simulink model "Motor_ctrl_INST"  (R2025b)
settings: Solver=ode15s  StartTime=0.0  StopTime=1  FixedStep=Ts/10  MaxStep=Tstep  RelTol=1e-3  AbsTol=1e-3  EnableMultiTasking=on
InitFcn:
  | if ~exist('flagwp')
  |     tic
  |     init_sim
  | end
  | mex Motor_ctrl.c User_functions/Src/*.c
StopFcn:
  | if ~exist('flagwp')
  |   elapsed_time=toc
  | end
values from neighbouring files (symbols this model uses):
  accel = 5000    [init_sim.m]
  Bm = 0    [init_sim.m]
  Clarke_inv = [1 0;-0.5 sqrt(3)/2;-0.5 -sqrt(3)/2]    [init_sim.m]
  Ctrl_strategy = 1    [init_sim.m]
  Ctrl_type = 3    [init_sim.m]
  dem = 1    [init_sim.m]
  dT = motorModel.SyreDrive.Converter.dT * 1e-6    [init_sim.m]
  expC = motorModel.IronPMLossMap_dq.expC    [init_sim.m]
  expH = motorModel.IronPMLossMap_dq.expH    [init_sim.m]
  expPM = motorModel.IronPMLossMap_dq.expPM    [init_sim.m]
  Fd0 = interp2(motorModel.FluxMap_dq.Id,motorModel.FluxMap_dq.Iq,motorModel.FluxMap_dq.Fd,0,0)    [init_sim.m]
  Fm = interp2(Idd,Iqq,Fdd,0,0)    [init_sim.m]
  HS_ctrl = 1    [init_sim.m]
  Id_dqt = interpn(motorModel.FluxMapInv_dqt.dataF.Fd,motorModel.FluxMapInv_dqt.dataF.Fq,motorModel.FluxMapInv_dqt.dataF.th,motorModel.FluxMapInv_dqt.dataF.Id,Fd_dqt,Fq_dqt,th_dqt,'cubic')    [init_sim.m]
  Id_fe = motorModel.IronPMLossMap_dq.Id    [init_sim.m]
  InitIntg_d = Fm*cos(th0)    [init_sim.m]
  InitIntg_q = Fm*sin(th0)    [init_sim.m]
  inj_waveform = 1    [init_sim.m]
  Iq_dqt = interpn(motorModel.FluxMapInv_dqt.dataF.Fd,motorModel.FluxMapInv_dqt.dataF.Fq,motorModel.FluxMapInv_dqt.dataF.th,motorModel.FluxMapInv_dqt.dataF.Iq,Fd_dqt,Fq_dqt,th_dqt,'cubic')    [init_sim.m]
  Iq_fe = motorModel.IronPMLossMap_dq.Iq    [init_sim.m]
  IronLoss = 1    [init_sim.m]
  J = motorModel.data.J    [init_sim.m]
  n0 = motorModel.IronPMLossMap_dq.n0    [init_sim.m]
  p = motorModel.data.p    [init_sim.m]
  Pfe_c = motorModel.IronPMLossMap_dq.Pfes_c + motorModel.IronPMLossMap_dq.Pfer_c    [init_sim.m]
  Pfe_h = motorModel.IronPMLossMap_dq.Pfes_h + motorModel.IronPMLossMap_dq.Pfer_h    [init_sim.m]
  Ppm = motorModel.IronPMLossMap_dq.Ppm    [init_sim.m]
  Quad_Maps = 2    [init_sim.m]
  SS_on = 1    [init_sim.m]
  T_dqt = interpn(motorModel.FluxMapInv_dqt.dataF.Fd,motorModel.FluxMapInv_dqt.dataF.Fq,motorModel.FluxMapInv_dqt.dataF.th,motorModel.FluxMapInv_dqt.dataF.T,Fd_dqt,Fq_dqt,th_dqt,'cubic')    [init_sim.m]
  Tf = 0    [init_sim.m]
  th0 = 0    [init_sim.m]
  th_max = max(motorModel.FluxMapInv_dqt.dataF.th,[],'all')    [init_sim.m]
  th_min = min(motorModel.FluxMapInv_dqt.dataF.th,[],'all')    [init_sim.m]
  Ts = 1/motorModel.SyreDrive.Converter.fPWM    [init_sim.m]
  Tv = 0    [init_sim.m]
  VDC = motorModel.data.Vdc    [init_sim.m]
undefined symbols (not defined in the file or in its folder): ACloss, eMotor, fD_pu_norm, fD_vct_max, fD_vct_ref, fQ_pu_norm, fQ_vct_max, fQ_vct_ref, iD_pu_norm, idRef, interpn, iQ_pu_norm, iqRef, J_rot, magnitude, motorModelType, nRef, sigbuilder_block, T0
libraries: nesl_utility x43, fl_lib x41, ee_lib x8, simulink x8, eeTransforms x1
(part 2 of 4)

== system Motor_ctrl_INST/Power block - Inverter + Motor/Circuital/Inverter Model/Inverter Commands/Duty ==
  Dabc : Inport
  iABC : Inport  Port=2
  Demux : Demux  Outputs=3
  Gain : Gain  Gain=dT/Ts
  Mux14 : Mux  Inputs=6
  Sign : Signum
  Sum : Sum  Inputs=|+-
  X_d1 : Fcn  Expr=1-u(1)
  X_d12 : Fcn  Expr=1-u(1)
  X_d2 : Fcn  Expr=1-u(1)
  G : Outport  VectorParamsAs1DForOutWhenUnconnected=off
  wires:
  iABC/1 -> Sign/1
  Sign/1 -> Gain/1
  Demux/3 -> Mux14/5, X_d2/1
  X_d2/1 -> Mux14/6
  Demux/1 -> X_d12/1, Mux14/1
  Dabc/1 -> Sum/1
  Gain/1 -> Sum/2
  Sum/1 -> Demux/1
  Demux/2 -> Mux14/3, X_d1/1
  X_d1/1 -> Mux14/4
  X_d12/1 -> Mux14/2
  Mux14/1 -> G/1

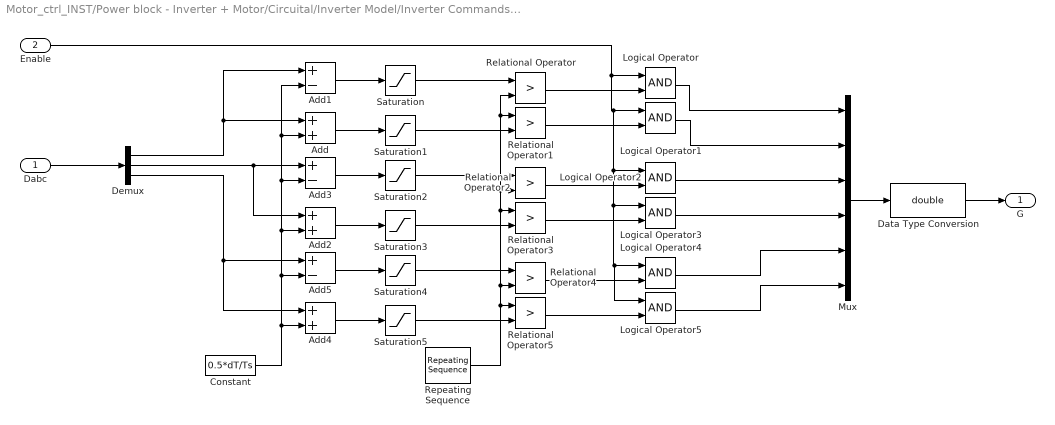
== system Motor_ctrl_INST/Power block - Inverter + Motor/Circuital/Inverter Model/Inverter Commands/PWM ==
  Dabc : Inport
  Enable : Inport  Port=2
  Add : Sum
  Add1 : Sum  Inputs=+-
  Add2 : Sum
  Add3 : Sum  Inputs=+-
  Add4 : Sum
  Add5 : Sum  Inputs=+-
  Constant : Constant  Value=0.5*dT/Ts
  Data Type Conversion : DataTypeConversion  OutDataTypeStr=double  SaturateOnIntegerOverflow=off  RndMeth=Floor
  Demux : Demux  Outputs=3
  Logical Operator{,1..5} (6 alike) : Logic  AllPortsSameDT=off  OutDataTypeStr=boolean
  Mux : Mux  Inputs=6
  Relational Operator{,1..5} (6 alike) : RelationalOperator  Operator=>  OutDataTypeStr=boolean  RndMeth=Simplest  InputSameDT=off
  Repeating Sequence : simulink/Sources/Repeating Sequence  rep_seq_t=[0 Ts/2 Ts]  rep_seq_y=[0 1 0]
  Saturation{,1..5} (6 alike) : Saturate  UpperLimit=1  LowerLimit=0
  G : Outport
  wires:
  Demux/3 -> Add4/1, Add5/1
  Add4/1 -> Saturation5/1
  Relational Operator4/1 -> Logical Operator4/2
  Add/1 -> Saturation1/1
  Relational Operator/1 -> Logical Operator/2
  Enable/1 -> Logical Operator5/1, Logical Operator4/1, Logical Operator3/1, Logical Operator2/1, Logical Operator1/1, Logical Operator/1
  Add5/1 -> Saturation4/1
  Relational Operator3/1 -> Logical Operator3/2
  Add1/1 -> Saturation/1
  Constant/1 -> Add1/2, Add/2, Add3/2, Add2/2, Add5/2, Add4/2
  Demux/1 -> Add1/1, Add/1
  Saturation2/1 -> Relational Operator2/1
  Demux/2 -> Add3/1, Add2/1
  Relational Operator2/1 -> Logical Operator2/2
  Saturation5/1 -> Relational Operator5/2
  Relational Operator1/1 -> Logical Operator1/2
  Add3/1 -> Saturation2/1
  Add2/1 -> Saturation3/1
  Saturation/1 -> Relational Operator/1
  Saturation4/1 -> Relational Operator4/1
  Saturation1/1 -> Relational Operator1/2
  Relational Operator5/1 -> Logical Operator5/2
  Logical Operator/1 -> Mux/1
  Saturation3/1 -> Relational Operator3/2
  Logical Operator1/1 -> Mux/2
  Dabc/1 -> Demux/1
  Mux/1 -> Data Type Conversion/1
  Logical Operator2/1 -> Mux/3
  Logical Operator3/1 -> Mux/4
  Logical Operator4/1 -> Mux/5
  Logical Operator5/1 -> Mux/6
  Repeating Sequence/1 -> Relational Operator/2, Relational Operator1/1, Relational Operator2/2, Relational Operator3/1, Relational Operator4/2, Relational Operator5/1
  Data Type Conversion/1 -> G/1

== system Motor_ctrl_INST/Power block - Inverter + Motor/Circuital/Motor model/CCG model/Mechanical equations ==
  Tload : Inport
  Tm : Inport  Port=2
  RPM : Inport  Port=3
  Constant : Constant  Value=Tf
  Constant1 : Constant  Value=Tv
  Delay One Step1 : Delay  DelayLength=1
  Delay One Step2 : Delay  DelayLength=1
  Gain1 : Gain  Gain=30/pi
  Gain2 : Gain  Gain=Bm  SaturateOnIntegerOverflow=on  OutDataTypeStr=Inherit: Same as input  ParamDataTypeStr=Inherit: Same as input
  Gain3 : Gain  Gain=1/J  SaturateOnIntegerOverflow=on  OutDataTypeStr=Inherit: Same as input  ParamDataTypeStr=Inherit: Same as input
  Gain4 : Gain  Gain=(2*pi)/60
  Integrator : Integrator  InitialCondition=th0  WrapState=on  WrappedStateUpperValue=2*pi  WrappedStateLowerValue=0
  Integrator1 : Integrator
  Integrator2 : Integrator  InitialCondition=th0  WrapState=on  WrappedStateUpperValue=2*pi  WrappedStateLowerValue=0
  Math Function1 : Math  Operator=magnitude^2  SignedPower=on
  Product : Product  SaturateOnIntegerOverflow=on  OutDataTypeStr=Inherit: Same as first input
  Product3 : Product  SaturateOnIntegerOverflow=on  OutDataTypeStr=Inherit: Same as first input
  Product6 : Product  SaturateOnIntegerOverflow=on  OutDataTypeStr=Inherit: Same as first input
  Sign : Signum  ZeroCross=off
  Sum1 : Sum  SaturateOnIntegerOverflow=on  OutDataTypeStr=Inherit: Same as first input
  Sum4 : Sum  SaturateOnIntegerOverflow=on  OutDataTypeStr=Inherit: Same as first input
  Sum5 : Sum  Inputs=--+  SaturateOnIntegerOverflow=on  OutDataTypeStr=Inherit: Same as first input
  Switch : Switch  Criteria=u2 > Threshold  Threshold=2.5  SaturateOnIntegerOverflow=off  InputSameDT=off
  Switch1 : Switch  Criteria=u2 > Threshold  Threshold=2.5  SaturateOnIntegerOverflow=off  InputSameDT=off
  n_m : Outport
  Pmec_out : Outport  Port=2  VectorParamsAs1DForOutWhenUnconnected=off
  thetar : Outport  Port=3
  wires:
  Gain3/1 -> Integrator1/1
  Gain2/1 -> Sum1/2
  Delay One Step2/1 -> Math Function1/1, Sign/1, Gain2/1
  Product6/1 -> Sum1/1
  Sum1/1 -> Sum5/2  "T mech loss"
  Tm/1 -> Delay One Step1/1
  Product/1 -> Pmec_out/1
  Tload/1 -> Sum5/1
  Math Function1/1 -> Product3/2
  Constant1/1 -> Product3/1
  Product3/1 -> Sum4/2
  Constant/1 -> Sum4/1
  Sum5/1 -> Gain3/1
  Sign/1 -> Product6/2
  Sum4/1 -> Product6/1
  Integrator2/1 -> Switch1/3
  Integrator/1 -> Switch1/1
  Switch1/1 -> thetar/1
  Switch/1 -> Gain1/1
  Integrator1/1 -> Integrator/1, Switch/1, Delay One Step2/1, Product/2
  Gain4/1 -> Switch/3, Integrator2/1
  [Ctrl_type] -> Switch/2, Switch1/2
  RPM/1 -> Gain4/1
  Delay One Step1/1 -> Sum5/3, Product/1
  Gain1/1 -> n_m/1

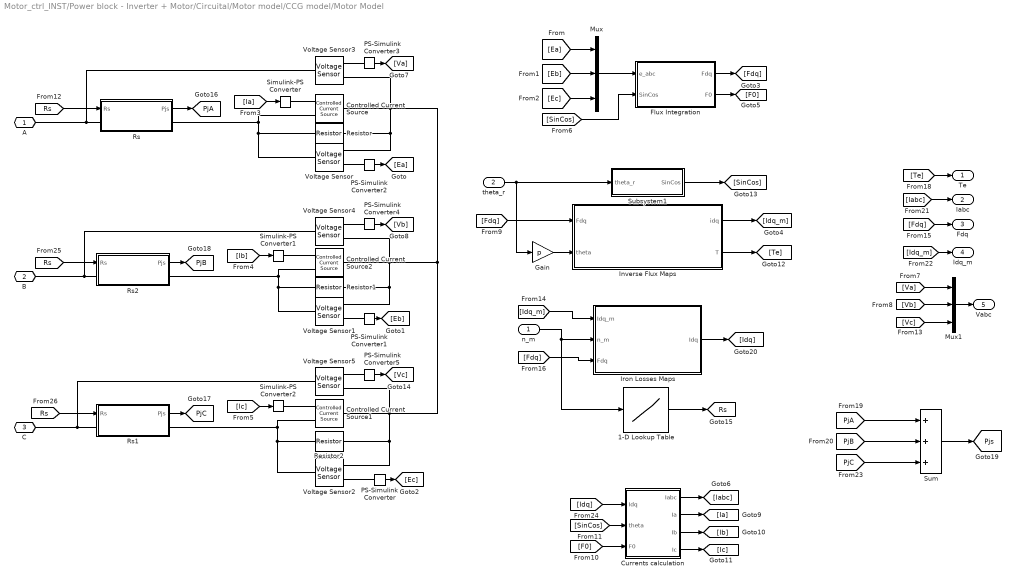
== system Motor_ctrl_INST/Power block - Inverter + Motor/Circuital/Motor model/CCG model/Motor Model ==
  n_m : Inport
  theta_r : Inport  Port=2
  1-D Lookup Table : Lookup_n-D  NumberOfTableDimensions=1  BreakpointsForDimension1=ACloss.n  Table=ACloss.Rac  InternalRulePriority=Speed  RndMeth=Simplest
  Controlled Current Source : fl_lib/Electrical/Electrical Sources/Controlled Current Source
  Controlled Current Source1 : fl_lib/Electrical/Electrical Sources/Controlled Current Source
  Controlled Current Source2 : fl_lib/Electrical/Electrical Sources/Controlled Current Source
  Currents calculation : Subsystem
  Flux Integration : Subsystem
  Gain : Gain  Gain=p
  Inverse Flux Maps : Subsystem  Variant=on
  Iron Losses Maps : Subsystem  Variant=on
  Mux : Mux  Inputs=3
  Mux1 : Mux  Inputs=3
  PS-Simulink Converter{,1..5} (6 alike) : nesl_utility/PS-Simulink Converter  PhysicalDomain=network_engine_domain  SubClassName=ps_output  LeftPortType=input  RightPortType=output  PseudoPeriodic=off  Frequencies=[]  VectorFormat=1-D array  Unit=inherit  AffineConversion=off
  Resistor : ee_lib/Passive/Resistor  R=1e9 Ohm  enable_R_tol=0  R_tol=5  tol_distribution=1  nSigma=4  enable_operating_limits=0  operating_limit_action=2  power_rating=1 W  max_working_voltage=100 V  noise_mode=0  Tdevice=25 degC  sample_time=1e-3 s  repeatability=1  user_seed=0  auto_seed=4111000739  power_derating_T1=70 degC  power_derating_T2=155 degC  operating_temperature_range_vec=[-50, 150] degC  alpha=3.93e-3 1/K  Tmeas=25 degC  thermal_mass=100 J/K  temperature_specify=off  temperature_priority=High  temperature=298.15 K  temperature_nominal_specify=off  temperature_nominal_value=1  temperature_nominal_unit=K
  Resistor1 : ee_lib/Passive/Resistor  R=1e9 Ohm  enable_R_tol=0  R_tol=5  tol_distribution=1  nSigma=4  enable_operating_limits=0  operating_limit_action=2  power_rating=1 W  max_working_voltage=100 V  noise_mode=0  Tdevice=25 degC  sample_time=1e-3 s  repeatability=1  user_seed=0  auto_seed=2084672538  power_derating_T1=70 degC  power_derating_T2=155 degC  operating_temperature_range_vec=[-50, 150] degC  alpha=3.93e-3 1/K  Tmeas=25 degC  thermal_mass=100 J/K  temperature_specify=off  temperature_priority=High  temperature=298.15 K  temperature_nominal_specify=off  temperature_nominal_value=1  temperature_nominal_unit=K
  Resistor2 : ee_lib/Passive/Resistor  R=1e9 Ohm  enable_R_tol=0  R_tol=5  tol_distribution=1  nSigma=4  enable_operating_limits=0  operating_limit_action=2  power_rating=1 W  max_working_voltage=100 V  noise_mode=0  Tdevice=25 degC  sample_time=1e-3 s  repeatability=1  user_seed=0  auto_seed=3437178441  power_derating_T1=70 degC  power_derating_T2=155 degC  operating_temperature_range_vec=[-50, 150] degC  alpha=3.93e-3 1/K  Tmeas=25 degC  thermal_mass=100 J/K  temperature_specify=off  temperature_priority=High  temperature=298.15 K  temperature_nominal_specify=off  temperature_nominal_value=1  temperature_nominal_unit=K
  Rs : Subsystem  Variant=on
  Rs1 : Subsystem  Variant=on
  Rs2 : Subsystem  Variant=on
  Simulink-PS Converter : nesl_utility/Simulink-PS Converter  PhysicalDomain=network_engine_domain  SubClassName=ps_input  LeftPortType=input  RightPortType=output  PseudoPeriodic=off  Frequencies=[]  NoiseDistribution=none  NoiseParameters=[]  Unit=1  AffineConversion=off  FilteringAndDerivatives=provide  SimscapeFilterOrder=1  InputFilterTimeConstant=0.001  UdotUserProvided=0
  Simulink-PS Converter1 : nesl_utility/Simulink-PS Converter  PhysicalDomain=network_engine_domain  SubClassName=ps_input  LeftPortType=input  RightPortType=output  PseudoPeriodic=off  Frequencies=[]  NoiseDistribution=none  NoiseParameters=[]  Unit=1  AffineConversion=off  FilteringAndDerivatives=provide  SimscapeFilterOrder=1  InputFilterTimeConstant=0.001  UdotUserProvided=0
  Simulink-PS Converter2 : nesl_utility/Simulink-PS Converter  PhysicalDomain=network_engine_domain  SubClassName=ps_input  LeftPortType=input  RightPortType=output  PseudoPeriodic=off  Frequencies=[]  NoiseDistribution=none  NoiseParameters=[]  Unit=1  AffineConversion=off  FilteringAndDerivatives=provide  SimscapeFilterOrder=1  InputFilterTimeConstant=0.001  UdotUserProvided=0
  Subsystem1 : Subsystem
  Sum : Sum  Inputs=+++
  Voltage Sensor{,1..5} (6 alike) : fl_lib/Electrical/Electrical Sensors/Voltage Sensor
  A : PMIOPort  Side=Left
  B : PMIOPort  Port=2  Side=Left
  C : PMIOPort  Port=3  Side=Left
  Te : Outport
  Iabc : Outport  Port=2
  Fdq : Outport  Port=3
  Idq_m : Outport  Port=4
  Vabc : Outport  Port=5
  tag scope: PjA=global, PjB=global, PjC=global, Pjs=global, Rs=global
  wires:
  PS-Simulink Converter2/1 -> [Ea]
  PS-Simulink Converter1/1 -> [Eb]
  PS-Simulink Converter/1 -> [Ec]
  [Ea] -> Mux/1
  [Eb] -> Mux/2
  [Ec] -> Mux/3
  [Ia] -> Simulink-PS Converter/1
  [Ib] -> Simulink-PS Converter1/1
  [Ic] -> Simulink-PS Converter2/1
  Inverse Flux Maps/1(idq) -> [Idq_m]
  [Iabc] -> Iabc/1
  [Idq_m] -> Idq_m/1
  [F0] -> Currents calculation/3(F0)
  [SinCos] -> Currents calculation/2(theta)
  [Idq] -> Currents calculation/1(Idq)
  [Fdq] -> Inverse Flux Maps/1(Fdq)
  [Te] -> Te/1
  theta_r/1 -> Gain/1, Subsystem1/1(theta_r)
  Currents calculation/1(Iabc) -> [Iabc]
  [Fdq] -> Fdq/1
  Subsystem1/1(SinCos) -> [SinCos]
  Mux/1 -> Flux Integration/1(e_abc)
  Flux Integration/1(Fdq) -> [Fdq]
  [SinCos] -> Flux Integration/2(SinCos)
  Flux Integration/2(F0) -> [F0]
  PS-Simulink Converter3/1 -> [Va]
  PS-Simulink Converter4/1 -> [Vb]
  PS-Simulink Converter5/1 -> [Vc]
  [Va] -> Mux1/1
  [Vb] -> Mux1/2
  [Vc] -> Mux1/3
  Mux1/1 -> Vabc/1
  Inverse Flux Maps/2(T) -> [Te]
  n_m/1 -> 1-D Lookup Table/1, Iron Losses Maps/2(n_m)
  [Fdq] -> Iron Losses Maps/3(Fdq)
  [Idq_m] -> Iron Losses Maps/1(Idq_m)
  Iron Losses Maps/1(Idq) -> [Idq]
  Currents calculation/2(Ia) -> [Ia]
  Currents calculation/3(Ib) -> [Ib]
  Currents calculation/4(Ic) -> [Ic]
  Gain/1 -> Inverse Flux Maps/2(theta)
  1-D Lookup Table/1 -> [Rs]
  [Rs] -> Rs/1(Rs)
  Rs/1(Pjs) -> [PjA]
  Rs2/1(Pjs) -> [PjB]
  Rs1/1(Pjs) -> [PjC]
  Sum/1 -> [Pjs]
  [PjC] -> Sum/3
  [PjB] -> Sum/2
  [PjA] -> Sum/1
  [Rs] -> Rs2/1(Rs)
  [Rs] -> Rs1/1(Rs)
  connections:
  Controlled Current Source/LConn1 -- Voltage Sensor3/RConn2 -- Voltage Sensor5/RConn2 -- Voltage Sensor2/RConn2 -- Resistor2/RConn1 -- Controlled Current Source1/LConn1 -- Voltage Sensor4/RConn2 -- Voltage Sensor1/RConn2 -- Resistor1/RConn1 -- Controlled Current Source2/LConn1 -- Voltage Sensor/RConn2 -- Resistor/RConn1
  Simulink-PS Converter/RConn1 -- Controlled Current Source/RConn1
  Simulink-PS Converter1/RConn1 -- Controlled Current Source2/RConn1
  Simulink-PS Converter2/RConn1 -- Controlled Current Source1/RConn1
  PS-Simulink Converter/LConn1 -- Voltage Sensor2/RConn1
  PS-Simulink Converter1/LConn1 -- Voltage Sensor1/RConn1
  PS-Simulink Converter2/LConn1 -- Voltage Sensor/RConn1
  Voltage Sensor2/LConn1 -- Resistor2/LConn1 -- Rs1/RConn1 -- Controlled Current Source1/RConn2
  Resistor1/LConn1 -- Rs2/RConn1 -- Controlled Current Source2/RConn2 -- Voltage Sensor1/LConn1
  Resistor/LConn1 -- Voltage Sensor/LConn1 -- Controlled Current Source/RConn2 -- Rs/RConn1
  Voltage Sensor3/LConn1 -- Rs/LConn1 -- A/RConn1
  Voltage Sensor4/LConn1 -- B/RConn1 -- Rs2/LConn1
  Voltage Sensor5/LConn1 -- Rs1/LConn1 -- C/RConn1
  Voltage Sensor3/RConn1 -- PS-Simulink Converter3/LConn1
  Voltage Sensor4/RConn1 -- PS-Simulink Converter4/LConn1
  Voltage Sensor5/RConn1 -- PS-Simulink Converter5/LConn1

== system Motor_ctrl_INST/Power block - Inverter + Motor/Circuital/Motor model/SimScape FEM-based PMSM/Load model ==
  note: 1) Add Subsystem or Model blocks as valid variant choices.
      | 2) You cannot connect blocks at this level. At simulation, connectivity is automatically
      | determined, based on the active variant and port name matching.
  T_ref : Inport
  n_ref : Inport  Port=2
  Ideal speed load : Subsystem  VariantControl=Ctrl_type<2.5
  Ideal torque load : Subsystem  VariantControl=Ctrl_type>2.5
  R : PMIOPort  Side=Left
  C : PMIOPort  Port=2  Side=Left

== system Motor_ctrl_INST/Power block - Inverter + Motor/Circuital/Motor model/SimScape FEM-based PMSM/abc2dq ==
  Xabc : Inport
  theta_r : Inport  Port=2
  Bus Creator : BusCreator  Inputs=2
  Demux : Demux  Outputs=3
  Subsystem1 : Subsystem
  Terminator : Terminator
  ab->dq : Subsystem
      mask Display: disp('A(-theta)')
  abc->ab0 : Subsystem
  X_dq : Outport
  wires:
  ab->dq/1(X_dq) -> X_dq/1
  Xabc/1 -> abc->ab0/1(eabc)
  Demux/1 -> Bus Creator/1
  Demux/2 -> Bus Creator/2
  abc->ab0/1(eab0) -> Demux/1
  Bus Creator/1 -> ab->dq/1(X_ab)
  Subsystem1/1(SinCos) -> ab->dq/2(sin,cos)
  theta_r/1 -> Subsystem1/1(theta_r)
  Demux/3 -> Terminator/1

== system Motor_ctrl_INST/Power block - Inverter + Motor/Circuital/Motor model/SimScape FEM-based PMSM/abc2dq1 ==
  Xabc : Inport
  theta_r : Inport  Port=2
  Bus Creator : BusCreator  Inputs=2
  Demux : Demux  Outputs=3
  Subsystem1 : Subsystem
  Terminator : Terminator
  ab->dq : Subsystem
      mask Display: disp('A(-theta)')
  abc->ab0 : Subsystem
  X_dq : Outport
  wires:
  ab->dq/1(X_dq) -> X_dq/1
  Xabc/1 -> abc->ab0/1(eabc)
  Demux/1 -> Bus Creator/1
  Demux/2 -> Bus Creator/2
  abc->ab0/1(eab0) -> Demux/1
  Bus Creator/1 -> ab->dq/1(X_ab)
  Subsystem1/1(SinCos) -> ab->dq/2(sin,cos)
  theta_r/1 -> Subsystem1/1(theta_r)
  Demux/3 -> Terminator/1

== system Motor_ctrl_INST/Power block - Inverter + Motor/Noncircuital/FM/Motor Model/Inverse Flux Maps ==
  note: 1) Add Subsystem or Model blocks as valid variant choices.
      | 2) You cannot connect blocks at this level. At simulation, connectivity is automatically
      | determined, based on the active variant and port name matching.
  Vabc : Inport
  theta_elt : Inport  Port=2
  n : Inport  Port=3
  2D LUT : Subsystem  VariantControl=FMapsModel==1
  3D LUTs : Subsystem  VariantControl=FMapsModel==-1
  idq : Outport
  T : Outport  Port=2
  i0 : Outport  Port=3
  Fdq : Outport  Port=4

== system Motor_ctrl_INST/Power block - Inverter + Motor/Noncircuital/FM/Motor Model/Iron Losses Maps ==
  note: 1) Add Subsystem or Model blocks as valid variant choices.
      | 2) You cannot connect blocks at this level. At simulation, connectivity is automatically
      | determined, based on the active variant and port name matching.
  Idq_m : Inport
  n_m : Inport  Port=2
  Fdq : Inport  Port=3
  T_m : Inport  Port=4
  Iron Losses : Subsystem  VariantControl=IronLoss==1
  No Iron Losses : Subsystem  VariantControl=IronLoss==0
  Idq : Outport

== system Motor_ctrl_INST/Power block - Inverter + Motor/Noncircuital/Inverter Model/Inverter Commands/Duty ==
  Dabc : Inport
  iABC : Inport  Port=2
  Gain : Gain  Gain=dT/Ts
  Gain1 : Gain  Gain=2*VDC/3
  Mux2 : Mux  Inputs=3
  Sign : Signum
  Sum : Sum  Inputs=|+-
  Unit Delay : UnitDelay  SampleTime=-1  HasFrameUpgradeWarning=on
  X_d6 : Fcn  Expr=-0.5*u(1) + u(2) - 0.5*u(3)
  X_d7 : Fcn  Expr=u(1) - 0.5*u(2) - 0.5*u(3)
  X_d8 : Fcn  Expr=-0.5*u(1) - 0.5*u(2) + u(3)
  Vabc : Outport  VectorParamsAs1DForOutWhenUnconnected=off
  wires:
  iABC/1 -> Sign/1
  Sign/1 -> Gain/1
  Dabc/1 -> Sum/1
  Gain/1 -> Sum/2
  Sum/1 -> Gain1/1
  X_d7/1 -> Mux2/1
  X_d6/1 -> Mux2/2
  X_d8/1 -> Mux2/3
  Unit Delay/1 -> Vabc/1
  Mux2/1 -> Unit Delay/1
  Gain1/1 -> X_d6/1, X_d8/1, X_d7/1

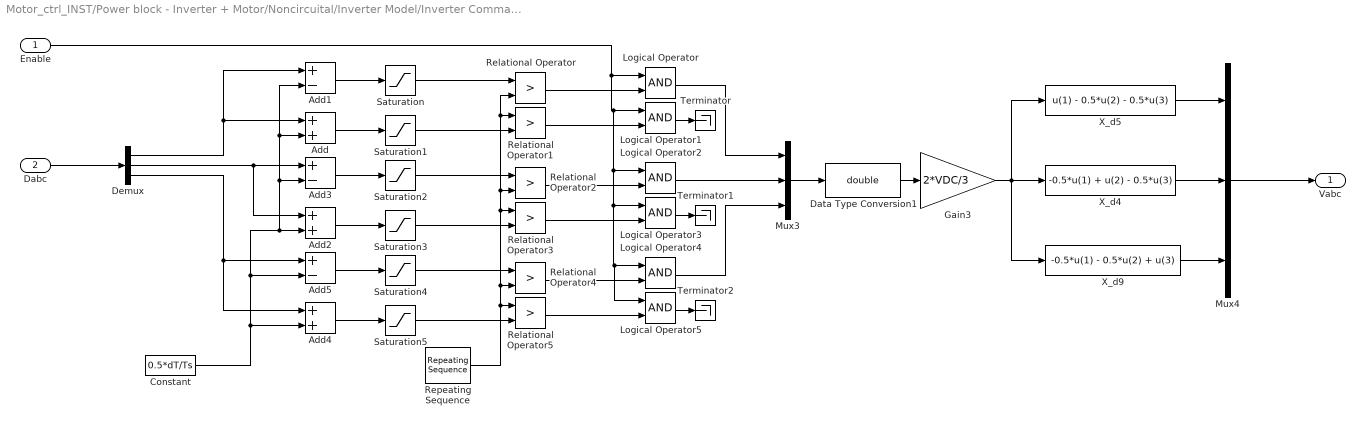
== system Motor_ctrl_INST/Power block - Inverter + Motor/Noncircuital/Inverter Model/Inverter Commands/PWM ==
  Enable : Inport
  Dabc : Inport  Port=2
  Add : Sum
  Add1 : Sum  Inputs=+-
  Add2 : Sum
  Add3 : Sum  Inputs=+-
  Add4 : Sum
  Add5 : Sum  Inputs=+-
  Constant : Constant  Value=0.5*dT/Ts
  Data Type Conversion1 : DataTypeConversion  OutDataTypeStr=double  SaturateOnIntegerOverflow=off  RndMeth=Floor
  Demux : Demux  Outputs=3
  Gain3 : Gain  Gain=2*VDC/3
  Logical Operator{,1..5} (6 alike) : Logic  AllPortsSameDT=off  OutDataTypeStr=boolean
  Mux3 : Mux  Inputs=3
  Mux4 : Mux  Inputs=3
  Relational Operator{,1..5} (6 alike) : RelationalOperator  Operator=>  OutDataTypeStr=boolean  RndMeth=Simplest  InputSameDT=off
  Repeating Sequence : simulink/Sources/Repeating Sequence  rep_seq_t=[0 Ts/2 Ts]  rep_seq_y=[0 1 0]
  Saturation{,1..5} (6 alike) : Saturate  UpperLimit=1  LowerLimit=0
  Terminator : Terminator
  Terminator1 : Terminator
  Terminator2 : Terminator
  X_d4 : Fcn  Expr=-0.5*u(1) + u(2) - 0.5*u(3)
  X_d5 : Fcn  Expr=u(1) - 0.5*u(2) - 0.5*u(3)
  X_d9 : Fcn  Expr=-0.5*u(1) - 0.5*u(2) + u(3)
  Vabc : Outport
  wires:
  Demux/3 -> Add4/1, Add5/1
  Add4/1 -> Saturation5/1
  Relational Operator4/1 -> Logical Operator4/2
  Add/1 -> Saturation1/1
  Relational Operator/1 -> Logical Operator/2
  Enable/1 -> Logical Operator5/1, Logical Operator4/1, Logical Operator3/1, Logical Operator2/1, Logical Operator1/1, Logical Operator/1
  Add5/1 -> Saturation4/1
  Relational Operator3/1 -> Logical Operator3/2
  Add1/1 -> Saturation/1
  Demux/1 -> Add1/1, Add/1
  Saturation2/1 -> Relational Operator2/1
  Demux/2 -> Add3/1, Add2/1
  Relational Operator2/1 -> Logical Operator2/2
  Saturation5/1 -> Relational Operator5/2
  Relational Operator1/1 -> Logical Operator1/2
  Add3/1 -> Saturation2/1
  Add2/1 -> Saturation3/1
  Saturation/1 -> Relational Operator/1
  Saturation4/1 -> Relational Operator4/1
  Saturation1/1 -> Relational Operator1/2
  Relational Operator5/1 -> Logical Operator5/2
  Logical Operator/1 -> Mux3/1
  Saturation3/1 -> Relational Operator3/2
  Logical Operator2/1 -> Mux3/2
  Logical Operator4/1 -> Mux3/3
  Repeating Sequence/1 -> Relational Operator/2, Relational Operator1/1, Relational Operator2/2, Relational Operator3/1, Relational Operator4/2, Relational Operator5/1
  X_d4/1 -> Mux4/2
  X_d5/1 -> Mux4/1
  X_d9/1 -> Mux4/3
  Gain3/1 -> X_d9/1, X_d5/1, X_d4/1
  Mux3/1 -> Data Type Conversion1/1
  Data Type Conversion1/1 -> Gain3/1
  Constant/1 -> Add1/2, Add/2, Add3/2, Add2/2, Add5/2, Add4/2
  Dabc/1 -> Demux/1
  Mux4/1 -> Vabc/1
  Logical Operator1/1 -> Terminator/1
  Logical Operator3/1 -> Terminator1/1
  Logical Operator5/1 -> Terminator2/1

== system Motor_ctrl_INST/Power block - Inverter + Motor/Circuital/Motor model/CCG model/Motor Model/Currents calculation ==
  Idq : Inport
  theta : Inport  Port=2
  F0 : Inport  Port=3
  2-->3 : Gain  Gain=Clarke_inv  Multiplication=Matrix(K*u)  SaturateOnIntegerOverflow=on  OutDataTypeStr=Inherit: Same as input  ParamDataTypeStr=Inherit: Same as input
  Demux : Demux  Outputs=3
  Demux1 : Demux  Outputs=3
  Gain1 : Gain  Gain=0
  Gain2 : Gain  Gain=1/3
  Mux3 : Mux  Inputs=3
  Sum1 : Sum  Inputs=|++
  Sum2 : Sum  Inputs=|++
  Sum3 : Sum  Inputs=|++
  dq->ab1 : Subsystem
      mask Display: disp('A(theta)')
  Iabc : Outport
  Ia : Outport  Port=2
  Ib : Outport  Port=3
  Ic : Outport  Port=4
  wires:
  Sum2/1 -> Mux3/2
  Demux1/3 -> Sum3/1
  2-->3/1 -> Demux1/1
  Demux1/1 -> Sum1/1
  Demux1/2 -> Sum2/1
  F0/1 -> Gain1/1
  Sum1/1 -> Mux3/1
  Sum3/1 -> Mux3/3
  Mux3/1 -> Demux/1, Iabc/1
  Gain1/1 -> Gain2/1
  Gain2/1 -> Sum1/2, Sum2/2, Sum3/2
  Idq/1 -> dq->ab1/1(X_ab)
  theta/1 -> dq->ab1/2(sin,cos)
  dq->ab1/1(X_dq) -> 2-->3/1
  Demux/1 -> Ia/1
  Demux/2 -> Ib/1
  Demux/3 -> Ic/1

== system Motor_ctrl_INST/Power block - Inverter + Motor/Circuital/Motor model/CCG model/Motor Model/Flux Integration ==
  e_abc : Inport
  SinCos : Inport  Port=2
  Demux : Demux  Outputs=3
  Demux1 : Demux  Outputs=3
  Integrator1 : Integrator  InitialCondition=InitIntg_d
  Integrator4 : Integrator  InitialCondition=InitIntg_q
  Integrator5 : Integrator
  Mux : Mux  Inputs=3
  Mux1 : Mux  Inputs=2
  ab->dq : Subsystem
      mask Display: disp('A(-theta)')
  abc->ab0 : Subsystem
  Fdq : Outport
  F0 : Outport  Port=2
  wires:
  Demux/3 -> Integrator5/1
  Demux/2 -> Integrator4/1
  Demux/1 -> Integrator1/1
  Integrator4/1 -> Mux/2
  Integrator1/1 -> Mux/1
  Integrator5/1 -> Mux/3
  e_abc/1 -> abc->ab0/1(eabc)
  abc->ab0/1(eab0) -> Demux/1
  Demux1/2 -> Mux1/2
  Mux1/1 -> ab->dq/1(X_ab)
  Demux1/1 -> Mux1/1
  ab->dq/1(X_dq) -> Fdq/1
  Demux1/3 -> F0/1
  SinCos/1 -> ab->dq/2(sin,cos)
  Mux/1 -> Demux1/1

== system Motor_ctrl_INST/Power block - Inverter + Motor/Circuital/Motor model/CCG model/Motor Model/Inverse Flux Maps ==
  note: 1) Add Subsystem or Model blocks as valid variant choices.
      | 2) You cannot connect blocks at this level. At simulation, connectivity is automatically
      | determined, based on the active variant and port name matching.
  Fdq : Inport
  theta : Inport  Port=2
  2D LUT : Subsystem  VariantControl=FMapsModel==1
  3D LUTs : Subsystem  VariantControl=FMapsModel==-1
  idq : Outport
  T : Outport  Port=2

== system Motor_ctrl_INST/Power block - Inverter + Motor/Circuital/Motor model/CCG model/Motor Model/Iron Losses Maps ==
  note: 1) Add Subsystem or Model blocks as valid variant choices.
      | 2) You cannot connect blocks at this level. At simulation, connectivity is automatically
      | determined, based on the active variant and port name matching.
  Idq_m : Inport
  n_m : Inport  Port=2
  Fdq : Inport  Port=3
  Iron Losses : Subsystem  VariantControl=IronLoss==1
  No Iron Losses : Subsystem  VariantControl=IronLoss==0
  Idq : Outport

== system Motor_ctrl_INST/Power block - Inverter + Motor/Circuital/Motor model/CCG model/Motor Model/Rs ==
  note: 1) Add Subsystem or Model blocks as valid variant choices.
      | 2) You cannot connect blocks at this level. At simulation, connectivity is automatically
      | determined, based on the active variant and port name matching.
  Rs : Inport
  no AC loss : Subsystem  VariantControl=ACloss.enable==0
  yes AC loss : Subsystem  VariantControl=ACloss.enable==1
  In : PMIOPort  Side=Left
  Out : PMIOPort  Port=2  Side=Right
  Pjs : Outport

== system Motor_ctrl_INST/Power block - Inverter + Motor/Circuital/Motor model/CCG model/Motor Model/Rs1 ==
  note: 1) Add Subsystem or Model blocks as valid variant choices.
      | 2) You cannot connect blocks at this level. At simulation, connectivity is automatically
      | determined, based on the active variant and port name matching.
  Rs : Inport
  no AC loss : Subsystem  VariantControl=ACloss.enable==0
  yes AC loss : Subsystem  VariantControl=ACloss.enable==1
  In : PMIOPort  Side=Left
  Out : PMIOPort  Port=2  Side=Right
  Pjs : Outport

== system Motor_ctrl_INST/Power block - Inverter + Motor/Circuital/Motor model/CCG model/Motor Model/Rs2 ==
  note: 1) Add Subsystem or Model blocks as valid variant choices.
      | 2) You cannot connect blocks at this level. At simulation, connectivity is automatically
      | determined, based on the active variant and port name matching.
  Rs : Inport
  no AC loss : Subsystem  VariantControl=ACloss.enable==0
  yes AC loss : Subsystem  VariantControl=ACloss.enable==1
  In : PMIOPort  Side=Left
  Out : PMIOPort  Port=2  Side=Right
  Pjs : Outport

== system Motor_ctrl_INST/Power block - Inverter + Motor/Circuital/Motor model/CCG model/Motor Model/Subsystem1 ==
  theta_r : Inport
  Gain1 : Gain  Gain=p
  Mux3 : Mux  Inputs=2
  Scope : Scope
  Scope1 : Scope
  Sin : Trigonometry
  Sin1 : Trigonometry  Operator=cos
  SinCos : Outport
  wires:
  Sin1/1 -> Mux3/2
  Sin/1 -> Mux3/1
  Mux3/1 -> Scope/1, SinCos/1
  Gain1/1 -> Scope1/1, Sin/1, Sin1/1
  theta_r/1 -> Gain1/1

== system Motor_ctrl_INST/Power block - Inverter + Motor/Circuital/Motor model/SimScape FEM-based PMSM/Load model/Ideal speed load ==
  T_ref : Inport
  n_ref : Inport  Port=2
  Gain : Gain  Gain=pi/30
  Ideal Angular Velocity Source : fl_lib/Mechanical/Mechanical Sources/Ideal Angular Velocity Source
  Simulink-PS Converter : nesl_utility/Simulink-PS Converter  PhysicalDomain=network_engine_domain  SubClassName=ps_input  LeftPortType=input  RightPortType=output  PseudoPeriodic=off  Frequencies=[]  NoiseDistribution=none  NoiseParameters=[]  Unit=1  AffineConversion=off  FilteringAndDerivatives=filter  SimscapeFilterOrder=1  InputFilterTimeConstant=0.001  UdotUserProvided=0
  Terminator : Terminator
  R : PMIOPort  Side=Left
  C : PMIOPort  Port=2  Side=Left
  wires:
  Gain/1 -> Simulink-PS Converter/1
  n_ref/1 -> Gain/1
  T_ref/1 -> Terminator/1
  connections:
  Ideal Angular Velocity Source/LConn1 -- R/RConn1
  Ideal Angular Velocity Source/RConn2 -- C/RConn1
  Simulink-PS Converter/RConn1 -- Ideal Angular Velocity Source/RConn1

== system Motor_ctrl_INST/Power block - Inverter + Motor/Circuital/Motor model/SimScape FEM-based PMSM/Load model/Ideal torque load ==
  T_ref : Inport
  n_ref : Inport  Port=2
  Ideal Torque Source : fl_lib/Mechanical/Mechanical Sources/Ideal Torque Source
  Simulink-PS Converter : nesl_utility/Simulink-PS Converter  PhysicalDomain=network_engine_domain  SubClassName=ps_input  LeftPortType=input  RightPortType=output  PseudoPeriodic=off  Frequencies=[]  NoiseDistribution=none  NoiseParameters=[]  Unit=1  AffineConversion=off  FilteringAndDerivatives=provide  SimscapeFilterOrder=1  InputFilterTimeConstant=0.001  UdotUserProvided=0
  Terminator : Terminator
  R : PMIOPort  Side=Left
  C : PMIOPort  Port=2  Side=Left
  wires:
  n_ref/1 -> Terminator/1
  T_ref/1 -> Simulink-PS Converter/1
  connections:
  Ideal Torque Source/LConn1 -- R/RConn1
  Ideal Torque Source/RConn2 -- C/RConn1
  Simulink-PS Converter/RConn1 -- Ideal Torque Source/RConn1

== system Motor_ctrl_INST/Power block - Inverter + Motor/Circuital/Motor model/SimScape FEM-based PMSM/abc2dq/Subsystem1 ==
  theta_r : Inport
  Gain1 : Gain  Gain=p
  Mux3 : Mux  Inputs=2
  Scope : Scope
  Scope1 : Scope
  Sin : Trigonometry
  Sin1 : Trigonometry  Operator=cos
  SinCos : Outport
  wires:
  Sin1/1 -> Mux3/2
  Sin/1 -> Mux3/1
  Mux3/1 -> Scope/1, SinCos/1
  Gain1/1 -> Scope1/1, Sin/1, Sin1/1
  theta_r/1 -> Gain1/1

== system Motor_ctrl_INST/Power block - Inverter + Motor/Circuital/Motor model/SimScape FEM-based PMSM/abc2dq/ab->dq ==
  X_ab : Inport
  sin,cos : Inport  Port=2
  Demux : Demux  Outputs=2
  Demux1 : Demux  Outputs=2
  Mux : Mux  Commented=on  Inputs=2
  Mux1 : Mux  Commented=on  Inputs=2
  Mux2 : Mux  Inputs=2
  Product{,1..3} (4 alike) : Product
  Subtract : Sum
  Subtract1 : Sum  Inputs=-+
  X_d : Fcn  Commented=on  Expr=u(1)*u(4) + u(2)*u(3)
  X_q : Fcn  Commented=on  Expr=- u(1)*u(3) + u(2)*u(4)
  X_dq : Outport  InitialOutput=0
  wires:
  X_q/1 -> Mux1/2
  X_d/1 -> Mux1/1
  Mux/1 -> X_q/1, X_d/1
  Demux1/2 -> Product1/2, Product/2
  Demux/2 -> Product1/1, Product2/1
  Demux1/1 -> Product3/2, Product2/2
  Product/1 -> Subtract/1
  Product2/1 -> Subtract/2
  Demux/1 -> Product3/1, Product/1
  Product3/1 -> Subtract1/1
  Product1/1 -> Subtract1/2
  Subtract/1 -> Mux2/1
  Subtract1/1 -> Mux2/2
  X_ab/1 -> Demux/1
  sin,cos/1 -> Demux1/1
  Mux2/1 -> X_dq/1

== system Motor_ctrl_INST/Power block - Inverter + Motor/Circuital/Motor model/SimScape FEM-based PMSM/abc2dq/abc->ab0 ==
  eabc : Inport
  Demux1 : Demux  Outputs=3
  Gain : Gain  Gain=0.5
  Gain1 : Gain  Gain=2/3
  Gain2 : Gain  Gain=1/sqrt(3)
  Gain3 : Gain  Gain=1/3
  Mux1 : Mux  Inputs=3
  Subtract : Sum  Inputs=+-
  Subtract1 : Sum
  Subtract2 : Sum  Inputs=+-
  Subtract3 : Sum  Inputs=+++
  eab0 : Outport
  wires:
  Subtract1/1 -> Gain/1
  Subtract/1 -> Gain1/1
  Demux1/2 -> Subtract3/2, Subtract2/1, Subtract1/1
  Subtract2/1 -> Gain2/1
  Subtract3/1 -> Gain3/1
  Gain1/1 -> Mux1/1
  Demux1/1 -> Subtract/1, Subtract3/1
  Gain3/1 -> Mux1/3
  Gain2/1 -> Mux1/2
  Gain/1 -> Subtract/2
  Mux1/1 -> eab0/1
  Demux1/3 -> Subtract3/3, Subtract2/2, Subtract1/2
  eabc/1 -> Demux1/1

== system Motor_ctrl_INST/Power block - Inverter + Motor/Circuital/Motor model/SimScape FEM-based PMSM/abc2dq1/Subsystem1 ==
  theta_r : Inport
  Gain1 : Gain  Gain=p
  Mux3 : Mux  Inputs=2
  Scope : Scope
  Scope1 : Scope
  Sin : Trigonometry
  Sin1 : Trigonometry  Operator=cos
  SinCos : Outport
  wires:
  Sin1/1 -> Mux3/2
  Sin/1 -> Mux3/1
  Mux3/1 -> Scope/1, SinCos/1
  Gain1/1 -> Scope1/1, Sin/1, Sin1/1
  theta_r/1 -> Gain1/1

== system Motor_ctrl_INST/Power block - Inverter + Motor/Circuital/Motor model/SimScape FEM-based PMSM/abc2dq1/ab->dq ==
  X_ab : Inport
  sin,cos : Inport  Port=2
  Demux : Demux  Outputs=2
  Demux1 : Demux  Outputs=2
  Mux : Mux  Commented=on  Inputs=2
  Mux1 : Mux  Commented=on  Inputs=2
  Mux2 : Mux  Inputs=2
  Product{,1..3} (4 alike) : Product
  Subtract : Sum
  Subtract1 : Sum  Inputs=-+
  X_d : Fcn  Commented=on  Expr=u(1)*u(4) + u(2)*u(3)
  X_q : Fcn  Commented=on  Expr=- u(1)*u(3) + u(2)*u(4)
  X_dq : Outport  InitialOutput=0
  wires:
  X_q/1 -> Mux1/2
  X_d/1 -> Mux1/1
  Mux/1 -> X_q/1, X_d/1
  Demux1/2 -> Product1/2, Product/2
  Demux/2 -> Product1/1, Product2/1
  Demux1/1 -> Product3/2, Product2/2
  Product/1 -> Subtract/1
  Product2/1 -> Subtract/2
  Demux/1 -> Product3/1, Product/1
  Product3/1 -> Subtract1/1
  Product1/1 -> Subtract1/2
  Subtract/1 -> Mux2/1
  Subtract1/1 -> Mux2/2
  X_ab/1 -> Demux/1
  sin,cos/1 -> Demux1/1
  Mux2/1 -> X_dq/1

== system Motor_ctrl_INST/Power block - Inverter + Motor/Circuital/Motor model/SimScape FEM-based PMSM/abc2dq1/abc->ab0 ==
  eabc : Inport
  Demux1 : Demux  Outputs=3
  Gain : Gain  Gain=0.5
  Gain1 : Gain  Gain=2/3
  Gain2 : Gain  Gain=1/sqrt(3)
  Gain3 : Gain  Gain=1/3
  Mux1 : Mux  Inputs=3
  Subtract : Sum  Inputs=+-
  Subtract1 : Sum
  Subtract2 : Sum  Inputs=+-
  Subtract3 : Sum  Inputs=+++
  eab0 : Outport
  wires:
  Subtract1/1 -> Gain/1
  Subtract/1 -> Gain1/1
  Demux1/2 -> Subtract3/2, Subtract2/1, Subtract1/1
  Subtract2/1 -> Gain2/1
  Subtract3/1 -> Gain3/1
  Gain1/1 -> Mux1/1
  Demux1/1 -> Subtract/1, Subtract3/1
  Gain3/1 -> Mux1/3
  Gain2/1 -> Mux1/2
  Gain/1 -> Subtract/2
  Mux1/1 -> eab0/1
  Demux1/3 -> Subtract3/3, Subtract2/2, Subtract1/2
  eabc/1 -> Demux1/1

== system Motor_ctrl_INST/Power block - Inverter + Motor/Noncircuital/FM/Motor Model/Inverse Flux Maps/2D LUT ==
  Vabc : Inport
  theta_elt : Inport  Port=2
  n : Inport  Port=3
  Gain : Gain  Gain=pi/30*p
  dq Model : Subsystem  Variant=on
  idq : Outport
  T : Outport  Port=2
  i0 : Outport  Port=3
  Fdq : Outport  Port=4
  wires:
  n/1 -> Gain/1
  Vabc/1 -> dq Model/1(Vabc)
  theta_elt/1 -> dq Model/2(theta_elt)
  dq Model/2(T) -> T/1
  Gain/1 -> dq Model/3(we)
  dq Model/1(idq) -> idq/1
  dq Model/3(i0) -> i0/1
  dq Model/4(Fdq) -> Fdq/1

== system Motor_ctrl_INST/Power block - Inverter + Motor/Noncircuital/FM/Motor Model/Inverse Flux Maps/3D LUTs ==
  Vabc : Inport
  theta_elt : Inport  Port=2
  n : Inport  Port=3
  Gain : Gain  Gain=pi/30*p
  Variant Subsystem : Subsystem  Variant=on
  idq : Outport
  T : Outport  Port=2
  i0 : Outport  Port=3
  Fdq : Outport  Port=4
  wires:
  Vabc/1 -> Variant Subsystem/1(Vabc)
  theta_elt/1 -> Variant Subsystem/2(theta_elt)
  Variant Subsystem/1(idq) -> idq/1
  Variant Subsystem/2(T) -> T/1
  n/1 -> Gain/1
  Gain/1 -> Variant Subsystem/3(we)
  Variant Subsystem/3(i0) -> i0/1
  Variant Subsystem/4(Fdq) -> Fdq/1

== system Motor_ctrl_INST/Power block - Inverter + Motor/Noncircuital/FM/Motor Model/Iron Losses Maps/Iron Losses ==
  Idq_m : Inport
  n_m : Inport  Port=2
  Fdq : Inport  Port=3
  Demux1 : Demux  Outputs=2
  Demux2 : Demux  Outputs=2
  Demux3 : Demux  Outputs=2
  Iron loss Maps : Subsystem
  Mux2 : Mux  Inputs=2
  Scope6 : Scope  NumInputPorts=2
  Sum1 : Sum  Inputs=|++
  Sum2 : Sum  Inputs=|++
  Idq : Outport
  tag scope: Ploss=global
  wires:
  Demux1/2 -> Sum2/1
  Sum2/1 -> Mux2/2
  Sum1/1 -> Mux2/1
  Demux1/1 -> Sum1/1
  Demux2/1 -> Sum1/2
  Demux2/2 -> Sum2/2
  Mux2/1 -> Idq/1
  Idq_m/1 -> Demux1/1, Iron loss Maps/1(Idq_m)
  n_m/1 -> Iron loss Maps/2(n_m)
  Fdq/1 -> Iron loss Maps/3(Fdq)
  Demux3/2 -> Scope6/2  "Iq_fe"
  Iron loss Maps/1(Idq_fe) -> Demux3/1, Demux2/1
  Demux3/1 -> Scope6/1  "Id_fe"
  Iron loss Maps/2(Ploss) -> [Ploss]

== system Motor_ctrl_INST/Power block - Inverter + Motor/Noncircuital/FM/Motor Model/Iron Losses Maps/No Iron Losses ==
  Idq_m : Inport
  Idq : Outport
  wires:
  Idq_m/1 -> Idq/1

== system Motor_ctrl_INST/Power block - Inverter + Motor/Circuital/Motor model/CCG model/Motor Model/Currents calculation/dq->ab1 ==
  X_ab : Inport
  sin,cos : Inport  Port=2
  Demux : Demux  Outputs=2
  Demux1 : Demux  Outputs=2
  Mux : Mux  Inputs=2
  Mux2 : Mux  Commented=on  Inputs=2
  Mux3 : Mux  Commented=on  Inputs=2
  Product{,1..3} (4 alike) : Product
  Subtract : Sum  Inputs=+-
  Subtract1 : Sum
  X_d1 : Fcn  Commented=on  Expr=u(1)*u(4) - u(2)*u(3)
  X_q1 : Fcn  Commented=on  Expr=u(1)*u(3) + u(2)*u(4)
  X_dq : Outport  InitialOutput=0
  wires:
  Mux3/1 -> X_d1/1, X_q1/1
  X_d1/1 -> Mux2/1
  X_q1/1 -> Mux2/2
  Demux/1 -> Product2/1, Product/1
  Demux1/2 -> Product3/2, Product/2
  Product1/1 -> Subtract/2
  Product/1 -> Subtract/1
  Demux/2 -> Product3/1, Product1/1
  Demux1/1 -> Product2/2, Product1/2
  Product2/1 -> Subtract1/1
  Product3/1 -> Subtract1/2
  Subtract/1 -> Mux/1
  Subtract1/1 -> Mux/2
  X_ab/1 -> Demux/1
  sin,cos/1 -> Demux1/1
  Mux/1 -> X_dq/1

== system Motor_ctrl_INST/Power block - Inverter + Motor/Circuital/Motor model/CCG model/Motor Model/Flux Integration/ab->dq ==
  X_ab : Inport
  sin,cos : Inport  Port=2
  Demux : Demux  Outputs=2
  Demux1 : Demux  Outputs=2
  Mux : Mux  Commented=on  Inputs=2
  Mux1 : Mux  Commented=on  Inputs=2
  Mux2 : Mux  Inputs=2
  Product{,1..3} (4 alike) : Product
  Subtract : Sum
  Subtract1 : Sum  Inputs=-+
  X_d : Fcn  Commented=on  Expr=u(1)*u(4) + u(2)*u(3)
  X_q : Fcn  Commented=on  Expr=- u(1)*u(3) + u(2)*u(4)
  X_dq : Outport  InitialOutput=0
  wires:
  X_q/1 -> Mux1/2
  X_d/1 -> Mux1/1
  Mux/1 -> X_q/1, X_d/1
  Demux1/2 -> Product1/2, Product/2
  Demux/2 -> Product1/1, Product2/1
  Demux1/1 -> Product3/2, Product2/2
  Product/1 -> Subtract/1
  Product2/1 -> Subtract/2
  Demux/1 -> Product3/1, Product/1
  Product3/1 -> Subtract1/1
  Product1/1 -> Subtract1/2
  Subtract/1 -> Mux2/1
  Subtract1/1 -> Mux2/2
  X_ab/1 -> Demux/1
  sin,cos/1 -> Demux1/1
  Mux2/1 -> X_dq/1

== system Motor_ctrl_INST/Power block - Inverter + Motor/Circuital/Motor model/CCG model/Motor Model/Flux Integration/abc->ab0 ==
  eabc : Inport
  Demux1 : Demux  Outputs=3
  Gain : Gain  Gain=0.5
  Gain1 : Gain  Gain=2/3
  Gain2 : Gain  Gain=1/sqrt(3)
  Gain3 : Gain  Gain=1/3
  Mux1 : Mux  Inputs=3
  Subtract : Sum  Inputs=+-
  Subtract1 : Sum
  Subtract2 : Sum  Inputs=+-
  Subtract3 : Sum  Inputs=+++
  eab0 : Outport
  wires:
  Subtract1/1 -> Gain/1
  Subtract/1 -> Gain1/1
  Demux1/2 -> Subtract3/2, Subtract2/1, Subtract1/1
  Subtract2/1 -> Gain2/1
  Subtract3/1 -> Gain3/1
  Gain1/1 -> Mux1/1
  Demux1/1 -> Subtract/1, Subtract3/1
  Gain3/1 -> Mux1/3
  Gain2/1 -> Mux1/2
  Gain/1 -> Subtract/2
  Mux1/1 -> eab0/1
  Demux1/3 -> Subtract3/3, Subtract2/2, Subtract1/2
  eabc/1 -> Demux1/1

== system Motor_ctrl_INST/Power block - Inverter + Motor/Circuital/Motor model/CCG model/Motor Model/Inverse Flux Maps/2D LUT ==
  Fdq : Inport
  dq Model : Subsystem  Variant=on
  idq : Outport
  T : Outport  Port=2
  wires:
  Fdq/1 -> dq Model/1(Fdq)
  dq Model/1(idq) -> idq/1
  dq Model/2(T) -> T/1

== system Motor_ctrl_INST/Power block - Inverter + Motor/Circuital/Motor model/CCG model/Motor Model/Inverse Flux Maps/3D LUTs ==
  Fdq : Inport
  theta : Inport  Port=2
  Variant Subsystem : Subsystem  Variant=on
  idq : Outport
  T : Outport  Port=2
  wires:
  Fdq/1 -> Variant Subsystem/1(Fdq)
  theta/1 -> Variant Subsystem/2(theta_elt)
  Variant Subsystem/1(idq) -> idq/1
  Variant Subsystem/2(T) -> T/1

== system Motor_ctrl_INST/Power block - Inverter + Motor/Circuital/Motor model/CCG model/Motor Model/Iron Losses Maps/Iron Losses ==
  Idq_m : Inport
  n_m : Inport  Port=2
  Fdq : Inport  Port=3
  Demux1 : Demux  Outputs=2
  Demux2 : Demux  Outputs=2
  Demux3 : Demux  Outputs=2
  Iron loss Maps : Subsystem
  Mux2 : Mux  Inputs=2
  Scope6 : Scope  NumInputPorts=2
  Sum1 : Sum  Inputs=|++
  Sum2 : Sum  Inputs=|++
  Idq : Outport
  tag scope: Ploss=global
  wires:
  Demux1/2 -> Sum2/1
  Sum2/1 -> Mux2/2
  Sum1/1 -> Mux2/1
  Demux1/1 -> Sum1/1
  Demux2/1 -> Sum1/2
  Demux2/2 -> Sum2/2
  Mux2/1 -> Idq/1
  Idq_m/1 -> Demux1/1, Iron loss Maps/1(Idq_m)
  n_m/1 -> Iron loss Maps/2(n_m)
  Fdq/1 -> Iron loss Maps/3(Fdq)
  Demux3/2 -> Scope6/2  "Iq_fe"
  Iron loss Maps/1(Idq_fe) -> Demux3/1, Demux2/1
  Demux3/1 -> Scope6/1  "Id_fe"
  Iron loss Maps/2(Ploss) -> [Ploss]

== system Motor_ctrl_INST/Power block - Inverter + Motor/Circuital/Motor model/CCG model/Motor Model/Iron Losses Maps/No Iron Losses ==
  Idq_m : Inport
  Idq : Outport
  wires:
  Idq_m/1 -> Idq/1

== system Motor_ctrl_INST/Power block - Inverter + Motor/Circuital/Motor model/CCG model/Motor Model/Rs/no AC loss ==
  Rs : Inport
  Current Sensor : fl_lib/Electrical/Electrical Sensors/Current Sensor
  PS-Simulink Converter : nesl_utility/PS-Simulink Converter  PhysicalDomain=network_engine_domain  SubClassName=ps_output  LeftPortType=input  RightPortType=output  PseudoPeriodic=off  Frequencies=[]  VectorFormat=inherit  Unit=inherit  AffineConversion=off
  PS-Simulink Converter1 : nesl_utility/PS-Simulink Converter  PhysicalDomain=network_engine_domain  SubClassName=ps_output  LeftPortType=input  RightPortType=output  PseudoPeriodic=off  Frequencies=[]  VectorFormat=inherit  Unit=inherit  AffineConversion=off
  Product : Product
  Resistor : fl_lib/Electrical/Electrical Elements/Resistor  R=ACloss.Rac(1) Ohm  i_specify=off  i_priority=None  i=0 A  i_nominal_specify=off  i_nominal_value=1  i_nominal_unit=A  v_specify=off  v_priority=None  v=0 V  v_nominal_specify=off  v_nominal_value=1  v_nominal_unit=V
  Terminator : Terminator
  Voltage Sensor : fl_lib/Electrical/Electrical Sensors/Voltage Sensor
  In : PMIOPort  Side=Left
  Out : PMIOPort  Port=2  Side=Right
  Pjs : Outport
  wires:
  PS-Simulink Converter/1 -> Product/1
  PS-Simulink Converter1/1 -> Product/2
  Product/1 -> Pjs/1
  Rs/1 -> Terminator/1
  connections:
  In/RConn1 -- Voltage Sensor/LConn1 -- Resistor/LConn1
  Current Sensor/RConn2 -- Out/RConn1
  Current Sensor/LConn1 -- Voltage Sensor/RConn2 -- Resistor/RConn1
  PS-Simulink Converter/LConn1 -- Voltage Sensor/RConn1
  PS-Simulink Converter1/LConn1 -- Current Sensor/RConn1

== system Motor_ctrl_INST/Power block - Inverter + Motor/Circuital/Motor model/CCG model/Motor Model/Rs/yes AC loss ==
  Rs : Inport
  Current Sensor : fl_lib/Electrical/Electrical Sensors/Current Sensor
  PS-Simulink Converter : nesl_utility/PS-Simulink Converter  PhysicalDomain=network_engine_domain  SubClassName=ps_output  LeftPortType=input  RightPortType=output  PseudoPeriodic=off  Frequencies=[]  VectorFormat=inherit  Unit=inherit  AffineConversion=off
  PS-Simulink Converter1 : nesl_utility/PS-Simulink Converter  PhysicalDomain=network_engine_domain  SubClassName=ps_output  LeftPortType=input  RightPortType=output  PseudoPeriodic=off  Frequencies=[]  VectorFormat=inherit  Unit=inherit  AffineConversion=off
  Product : Product
  Simulink-PS Converter : nesl_utility/Simulink-PS Converter  PhysicalDomain=network_engine_domain  SubClassName=ps_input  LeftPortType=input  RightPortType=output  PseudoPeriodic=off  Frequencies=[]  NoiseDistribution=none  NoiseParameters=[]  Unit=1  AffineConversion=off  FilteringAndDerivatives=provide  SimscapeFilterOrder=1  InputFilterTimeConstant=0.001  UdotUserProvided=0
  Variable Resistor : fl_lib/Electrical/Electrical Elements/Variable Resistor  Rmin=0 Ohm  thermalEnable=false  thermal_mass=1 J/K  i_specify=off  i_priority=None  i=0 A  i_nominal_specify=off  i_nominal_value=1  i_nominal_unit=A  v_specify=off  v_priority=None  v=0 V  v_nominal_specify=off  v_nominal_value=1  v_nominal_unit=V  T_specify=off  T_priority=None  T=300 K  T_nominal_specify=off  T_nominal_value=1  T_nominal_unit=K
  Voltage Sensor : fl_lib/Electrical/Electrical Sensors/Voltage Sensor
  In : PMIOPort  Side=Left
  Out : PMIOPort  Port=2  Side=Right
  Pjs : Outport
  wires:
  PS-Simulink Converter1/1 -> Product/2
  PS-Simulink Converter/1 -> Product/1
  Product/1 -> Pjs/1
  Rs/1 -> Simulink-PS Converter/1
  connections:
  Current Sensor/LConn1 -- Voltage Sensor/RConn2 -- Variable Resistor/RConn1
  In/RConn1 -- Variable Resistor/LConn2 -- Voltage Sensor/LConn1
  Current Sensor/RConn2 -- Out/RConn1
  PS-Simulink Converter1/LConn1 -- Current Sensor/RConn1
  PS-Simulink Converter/LConn1 -- Voltage Sensor/RConn1
  Variable Resistor/LConn1 -- Simulink-PS Converter/RConn1

== system Motor_ctrl_INST/Power block - Inverter + Motor/Circuital/Motor model/CCG model/Motor Model/Rs1/no AC loss ==
  Rs : Inport
  Current Sensor : fl_lib/Electrical/Electrical Sensors/Current Sensor
  PS-Simulink Converter : nesl_utility/PS-Simulink Converter  PhysicalDomain=network_engine_domain  SubClassName=ps_output  LeftPortType=input  RightPortType=output  PseudoPeriodic=off  Frequencies=[]  VectorFormat=inherit  Unit=inherit  AffineConversion=off
  PS-Simulink Converter1 : nesl_utility/PS-Simulink Converter  PhysicalDomain=network_engine_domain  SubClassName=ps_output  LeftPortType=input  RightPortType=output  PseudoPeriodic=off  Frequencies=[]  VectorFormat=inherit  Unit=inherit  AffineConversion=off
  Product : Product
  Resistor : fl_lib/Electrical/Electrical Elements/Resistor  R=ACloss.Rac(1) Ohm  i_specify=off  i_priority=None  i=0 A  i_nominal_specify=off  i_nominal_value=1  i_nominal_unit=A  v_specify=off  v_priority=None  v=0 V  v_nominal_specify=off  v_nominal_value=1  v_nominal_unit=V
  Terminator : Terminator
  Voltage Sensor : fl_lib/Electrical/Electrical Sensors/Voltage Sensor
  In : PMIOPort  Side=Left
  Out : PMIOPort  Port=2  Side=Right
  Pjs : Outport
  wires:
  PS-Simulink Converter/1 -> Product/1
  PS-Simulink Converter1/1 -> Product/2
  Product/1 -> Pjs/1
  Rs/1 -> Terminator/1
  connections:
  Resistor/LConn1 -- In/RConn1 -- Voltage Sensor/LConn1
  Current Sensor/RConn2 -- Out/RConn1
  Resistor/RConn1 -- Current Sensor/LConn1 -- Voltage Sensor/RConn2
  PS-Simulink Converter/LConn1 -- Voltage Sensor/RConn1
  PS-Simulink Converter1/LConn1 -- Current Sensor/RConn1

== system Motor_ctrl_INST/Power block - Inverter + Motor/Circuital/Motor model/CCG model/Motor Model/Rs1/yes AC loss ==
  Rs : Inport
  Current Sensor : fl_lib/Electrical/Electrical Sensors/Current Sensor
  PS-Simulink Converter : nesl_utility/PS-Simulink Converter  PhysicalDomain=network_engine_domain  SubClassName=ps_output  LeftPortType=input  RightPortType=output  PseudoPeriodic=off  Frequencies=[]  VectorFormat=inherit  Unit=inherit  AffineConversion=off
  PS-Simulink Converter1 : nesl_utility/PS-Simulink Converter  PhysicalDomain=network_engine_domain  SubClassName=ps_output  LeftPortType=input  RightPortType=output  PseudoPeriodic=off  Frequencies=[]  VectorFormat=inherit  Unit=inherit  AffineConversion=off
  Product : Product
  Simulink-PS Converter : nesl_utility/Simulink-PS Converter  PhysicalDomain=network_engine_domain  SubClassName=ps_input  LeftPortType=input  RightPortType=output  PseudoPeriodic=off  Frequencies=[]  NoiseDistribution=none  NoiseParameters=[]  Unit=1  AffineConversion=off  FilteringAndDerivatives=provide  SimscapeFilterOrder=1  InputFilterTimeConstant=0.001  UdotUserProvided=0
  Variable Resistor : fl_lib/Electrical/Electrical Elements/Variable Resistor  Rmin=0 Ohm  thermalEnable=false  thermal_mass=1 J/K  i_specify=off  i_priority=None  i=0 A  i_nominal_specify=off  i_nominal_value=1  i_nominal_unit=A  v_specify=off  v_priority=None  v=0 V  v_nominal_specify=off  v_nominal_value=1  v_nominal_unit=V  T_specify=off  T_priority=None  T=300 K  T_nominal_specify=off  T_nominal_value=1  T_nominal_unit=K
  Voltage Sensor : fl_lib/Electrical/Electrical Sensors/Voltage Sensor
  In : PMIOPort  Side=Left
  Out : PMIOPort  Port=2  Side=Right
  Pjs : Outport
  wires:
  PS-Simulink Converter1/1 -> Product/2
  PS-Simulink Converter/1 -> Product/1
  Product/1 -> Pjs/1
  Rs/1 -> Simulink-PS Converter/1
  connections:
  Variable Resistor/RConn1 -- Current Sensor/LConn1 -- Voltage Sensor/RConn2
  In/RConn1 -- Voltage Sensor/LConn1 -- Variable Resistor/LConn2
  Current Sensor/RConn2 -- Out/RConn1
  PS-Simulink Converter1/LConn1 -- Current Sensor/RConn1
  PS-Simulink Converter/LConn1 -- Voltage Sensor/RConn1
  Variable Resistor/LConn1 -- Simulink-PS Converter/RConn1
